simulink model "cascadeHbridge"  (R2024a)
settings: Solver=VariableStepAuto  StartTime=0.0  StopTime=1  RelTol=1e-3
libraries: spsIGBTDiodeLib x24, spsTriangleGeneratorLib x12, spsDCVoltageSourceLib x6, spsSeriesRLCBranchLib x3, spsGroundLib x2, spsThreePhaseVIMeasurementLib x1, sps_lib x1
settings Model: Creator=SAI DEEPAK  LastModifiedBy=SAI DEEPAK
settings DataIOCC: ReturnWorkspaceOutputs=off

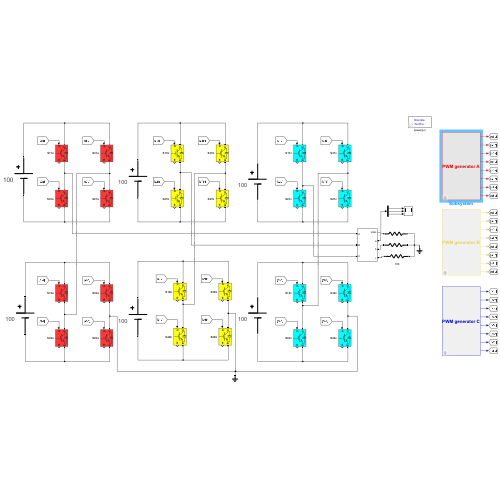
[thumbnail: Simulink's stored preview of the top-level diagram]
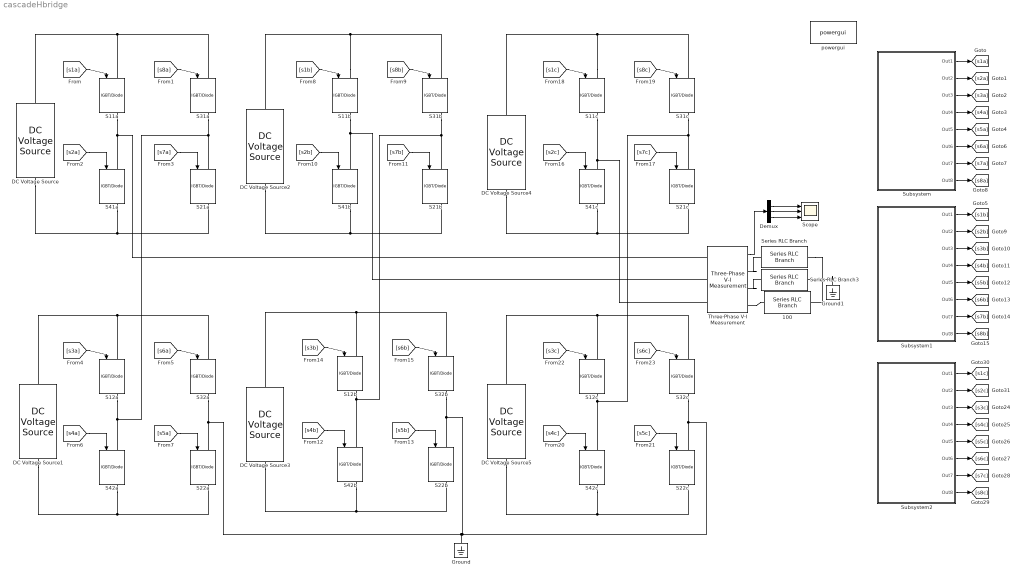
== system cascadeHbridge ==
  100 : spsSeriesRLCBranchLib/Series RLC Branch  LConnTagsString=__new0  RConnTagsString=__new0  BranchType=R  Resistance=100  Inductance=1e-3  SetiL0=off  InitialCurrent=0  Capacitance=1e-6  Setx0=off  InitialVoltage=0  Measurements=None
  DC Voltage Source{,1..5} (6 alike) : spsDCVoltageSourceLib/DC Voltage Source  Amplitude=100  Measurements=None
      settings: AttributesFormatString=%<Amplitude>
  Demux : Demux  Outputs=3
  Ground : spsGroundLib/Ground  LConnTagsString=a
  Ground1 : spsGroundLib/Ground  LConnTagsString=a
  S11a : spsIGBTDiodeLib/IGBT//Diode  Ron=1e-3  Rs=1e5  Cs=inf  Measurements=on
  S11b : spsIGBTDiodeLib/IGBT//Diode  Ron=1e-3  Rs=1e5  Cs=inf  Measurements=on
  S11c : spsIGBTDiodeLib/IGBT//Diode  Ron=1e-3  Rs=1e5  Cs=inf  Measurements=on
  S12a : spsIGBTDiodeLib/IGBT//Diode  Ron=1e-3  Rs=1e5  Cs=inf  Measurements=on
  S12b : spsIGBTDiodeLib/IGBT//Diode  Ron=1e-3  Rs=1e5  Cs=inf  Measurements=on
  S12c : spsIGBTDiodeLib/IGBT//Diode  Ron=1e-3  Rs=1e5  Cs=inf  Measurements=on
  S21a : spsIGBTDiodeLib/IGBT//Diode  Ron=1e-3  Rs=1e5  Cs=inf  Measurements=on
  S21b : spsIGBTDiodeLib/IGBT//Diode  Ron=1e-3  Rs=1e5  Cs=inf  Measurements=on
  S21c : spsIGBTDiodeLib/IGBT//Diode  Ron=1e-3  Rs=1e5  Cs=inf  Measurements=on
  S22a : spsIGBTDiodeLib/IGBT//Diode  Ron=1e-3  Rs=1e5  Cs=inf  Measurements=on
  S22b : spsIGBTDiodeLib/IGBT//Diode  Ron=1e-3  Rs=1e5  Cs=inf  Measurements=on
  S22c : spsIGBTDiodeLib/IGBT//Diode  Ron=1e-3  Rs=1e5  Cs=inf  Measurements=on
  S31a : spsIGBTDiodeLib/IGBT//Diode  Ron=1e-3  Rs=1e5  Cs=inf  Measurements=on
  S31b : spsIGBTDiodeLib/IGBT//Diode  Ron=1e-3  Rs=1e5  Cs=inf  Measurements=on
  S31c : spsIGBTDiodeLib/IGBT//Diode  Ron=1e-3  Rs=1e5  Cs=inf  Measurements=on
  S32a : spsIGBTDiodeLib/IGBT//Diode  Ron=1e-3  Rs=1e5  Cs=inf  Measurements=on
  S32b : spsIGBTDiodeLib/IGBT//Diode  Ron=1e-3  Rs=1e5  Cs=inf  Measurements=on
  S32c : spsIGBTDiodeLib/IGBT//Diode  Ron=1e-3  Rs=1e5  Cs=inf  Measurements=on
  S41a : spsIGBTDiodeLib/IGBT//Diode  Ron=1e-3  Rs=1e5  Cs=inf  Measurements=on
  S41b : spsIGBTDiodeLib/IGBT//Diode  Ron=1e-3  Rs=1e5  Cs=inf  Measurements=on
  S41c : spsIGBTDiodeLib/IGBT//Diode  Ron=1e-3  Rs=1e5  Cs=inf  Measurements=on
  S42a : spsIGBTDiodeLib/IGBT//Diode  Ron=1e-3  Rs=1e5  Cs=inf  Measurements=on
  S42b : spsIGBTDiodeLib/IGBT//Diode  Ron=1e-3  Rs=1e5  Cs=inf  Measurements=on
  S42c : spsIGBTDiodeLib/IGBT//Diode  Ron=1e-3  Rs=1e5  Cs=inf  Measurements=on
  Scope : Scope  NumInputPorts=3
  Series RLC Branch : spsSeriesRLCBranchLib/Series RLC Branch  LConnTagsString=__new0  RConnTagsString=__new0  BranchType=R  Resistance=100  Inductance=1e-3  SetiL0=off  InitialCurrent=0  Capacitance=1e-6  Setx0=off  InitialVoltage=0  Measurements=None
  Series RLC Branch3 : spsSeriesRLCBranchLib/Series RLC Branch  LConnTagsString=__new0  RConnTagsString=__new0  BranchType=R  Resistance=100  Inductance=1e-3  SetiL0=off  InitialCurrent=0  Capacitance=1e-6  Setx0=off  InitialVoltage=0  Measurements=None
  Subsystem : Subsystem  mask{Amplitude=0.8, Frequency=2*pi*50, Phaseangle=0, Freq1=2e3, Phase1=0, Freq2=2e3, Phase2=270, Freq3=2e3, Phase3=180, Freq4=2e3, Phase4=90}
      mask prompts: Amplitude "Simulink:blkprm_prompts:SinWaveAmplitude"; Frequency "Simulink:blkprm_prompts:SinWaveFrequency"; Phaseangle "Simulink:blkprm_prompts:SinWavePhase"; Freq1 "Frequency (Hz):"; Phase1 "Phase (degrees):"; Freq2 "Frequency (Hz):"; Phase2 "Phase (degrees):"; Freq3 "Frequency (Hz):"; Phase3 "Phase (degrees):"; Freq4 "Frequency (Hz):"; Phase4 "Phase (degrees):"
      mask TypeOptions Amplitude: Sine Wave/Amplitude
      mask TypeOptions Frequency: Sine Wave/Frequency
      mask TypeOptions Phaseangle: Sine Wave/Phase
      mask TypeOptions Freq1:
      | Triangle
      | Generator1/Freq
      mask TypeOptions Phase1:
      | Triangle
      | Generator1/Phase
      mask TypeOptions Freq2:
      | Triangle
      | Generator2/Freq
      mask TypeOptions Phase2:
      | Triangle
      | Generator2/Phase
      mask TypeOptions Freq3:
      | Triangle
      | Generator3/Freq
      mask TypeOptions Phase3:
      | Triangle
      | Generator3/Phase
      mask TypeOptions Freq4:
      | Triangle
      | Generator4/Freq
      mask TypeOptions Phase4:
      | Triangle
      | Generator4/Phase
      mask DialogControl Sinewave Prompt: (Add text here)
      mask DialogControl Amplitude Prompt: Amplitude:
      mask DialogControl Frequency Prompt: Frequency (rad/sec):
      mask DialogControl Phaseangle Prompt: Phase (rad):
      mask DialogControl carriersignal1 Prompt: (Add text here)
      mask DialogControl carriersignal2 Prompt: (Add text here)
      mask DialogControl carriersignal3 Prompt: (Add text here)
      mask DialogControl carriersignal4 Prompt: (Add text here)
      mask Display:
      | color('red');
      | disp('PWM generator A');
  Subsystem1 : Subsystem  mask{Amplitude=0.8, Frequency=2*pi*50, Phase=-2*pi/3, Freq1=2e3, Phase1=0, Freq2=2e3, Phase2=270, Freq3=2e3, Phase3=180, Freq4=2e3, Phase4=90}
      mask prompts: Amplitude "Simulink:blkprm_prompts:SinWaveAmplitude"; Frequency "Simulink:blkprm_prompts:SinWaveFrequency"; Phase "Simulink:blkprm_prompts:SinWavePhase"; Freq1 "Frequency (Hz):"; Phase1 "Phase (degrees):"; Freq2 "Frequency (Hz):"; Phase2 "Phase (degrees):"; Freq3 "Frequency (Hz):"; Phase3 "Phase (degrees):"; Freq4 "Frequency (Hz):"; Phase4 "Phase (degrees):"
      mask TypeOptions Amplitude: Sine Wave1/Amplitude
      mask TypeOptions Frequency: Sine Wave1/Frequency
      mask TypeOptions Phase: Sine Wave1/Phase
      mask TypeOptions Freq1:
      | Triangle
      | Generator4/Freq
      mask TypeOptions Phase1:
      | Triangle
      | Generator4/Phase
      mask TypeOptions Freq2:
      | Triangle
      | Generator5/Freq
      mask TypeOptions Phase2:
      | Triangle
      | Generator5/Phase
      mask TypeOptions Freq3:
      | Triangle
      | Generator6/Freq
      mask TypeOptions Phase3:
      | Triangle
      | Generator6/Phase
      mask TypeOptions Freq4:
      | Triangle
      | Generator7/Freq
      mask TypeOptions Phase4:
      | Triangle
      | Generator7/Phase
      mask DialogControl Control6 Prompt: modulating signal
      mask DialogControl Amplitude Prompt: Amplitude:
      mask DialogControl Frequency Prompt: Frequency (rad/sec):
      mask DialogControl Phase Prompt: Phase (rad):
      mask DialogControl Control1 Prompt: carrier signal 1
      mask DialogControl Control4 Prompt: carrier signal 2
      mask DialogControl Control3 Prompt: carrier signal 3
      mask DialogControl Control2 Prompt: carrier signal 4
      mask Display:
      | color('yellow');
      | disp('PWM generator B');
  Subsystem2 : Subsystem  mask{Amplitude=0.8, Frequency=2*pi*50, Phase=2*pi/3, Freq1=2e3, Phase1=0, Phase2=90, Freq2=2e3, Freq3=2e3, Phase3=180, Phase4=270, Freq4=2e3}
      mask prompts: Amplitude "Simulink:blkprm_prompts:SinWaveAmplitude"; Frequency "Simulink:blkprm_prompts:SinWaveFrequency"; Phase "Simulink:blkprm_prompts:SinWavePhase"; Freq1 "Frequency (Hz):"; Phase1 "Phase (degrees):"; Phase2 "Phase (degrees):"; Freq2 "Frequency (Hz):"; Freq3 "Frequency (Hz):"; Phase3 "Phase (degrees):"; Phase4 "Phase (degrees):"; Freq4 "Frequency (Hz):"
      mask TypeOptions Amplitude: Sine Wave3/Amplitude
      mask TypeOptions Frequency: Sine Wave3/Frequency
      mask TypeOptions Phase: Sine Wave3/Phase
      mask TypeOptions Freq1:
      | Triangle
      | Generator14/Freq
      mask TypeOptions Phase1:
      | Triangle
      | Generator14/Phase
      mask TypeOptions Phase2:
      | Triangle
      | Generator13/Phase
      mask TypeOptions Freq2:
      | Triangle
      | Generator13/Freq
      mask TypeOptions Freq3:
      | Triangle
      | Generator12/Freq
      mask TypeOptions Phase3:
      | Triangle
      | Generator12/Phase
      mask TypeOptions Phase4:
      | Triangle
      | Generator15/Phase
      mask TypeOptions Freq4:
      | Triangle
      | Generator15/Freq
      mask DialogControl Control2 Prompt: modulating signal
      mask DialogControl Amplitude Prompt: Amplitude:
      mask DialogControl Frequency Prompt: Frequency (rad/sec):
      mask DialogControl Phase Prompt: Phase (rad):
      mask DialogControl Control4 Prompt: carrier signal 1
      mask DialogControl Control5 Prompt: carrier signal 2
      mask DialogControl Control3 Prompt: carrier signal3
      mask DialogControl Control6 Prompt: carrier signal4
      mask Display:
      | color('blue');
      | disp('PWM generator C');
  Three-Phase V-I Measurement : spsThreePhaseVIMeasurementLib/Three-Phase V-I Measurement  VoltageMeasurement=phase-to-ground  SetLabelV=off  LabelV=Vabc  Vpu=off  VpuLL=off  CurrentMeasurement=no  SetLabelI=off  LabelI=Iabc  Ipu=off  Pbase=100e6  Vbase=500e3  OutputType=Complex  PhasorSimulation=off  PSBequivalent=0
  powergui : sps_lib/powergui  Priority=1  SimulationMode=Discrete  SampleTime=5e-6  frequency=60  Iterations=50  frequencyindice=0  Pbase=100e6  ErrMax=1e-4  UnitsV=kV  UnitsW=MW  buscounter=0  FunctionMessages=off  echomessages=off  EnableUseOfTLC=off  CurrentSourceSwitches=off  DisableSnubberDevices=off  DisableRonSwitches=off  DisableVfSwitches=off  DisplayEquations=off  AutomaticDiscreteSolvers=off  SolverType=Tustin/Backward Euler (TBE)  Interpol=off  ExternalGateDelay=off  methode=off  Ts=100  x0status=blocks  SPID=on  SwTol=0  HookPort=off  NonlinearTolerance=1e-4  nMaxIteration=100  ContinueOnMaxIteration=off  RestoreLinks=warning  ResistiveCurrentMeasurement=off  Frange=[0:2:500]  Ylog=off  Xlog=on  ShowGrid=off  save=off  variable=ZData  structure=0  ZoomFFT=off  StartTime=0.0  cycles=1  DisplayStyle=1  fundamental=60  FreqAxis=off  MaxFrequency=1000  frequencyindicesteady=1  RmsSteady=1  display=off
  wires:
  [s1a] -> S11a/1
  [s2a] -> S41a/1
  [s8a] -> S31a/1
  [s7a] -> S21a/1
  [s3a] -> S12a/1
  [s4a] -> S42a/1
  [s6a] -> S32a/1
  [s5a] -> S22a/1
  [s1b] -> S11b/1
  [s2b] -> S41b/1
  [s8b] -> S31b/1
  [s7b] -> S21b/1
  [s6b] -> S32b/1
  [s3b] -> S12b/1
  [s4b] -> S42b/1
  [s5b] -> S22b/1
  [s1c] -> S11c/1
  [s2c] -> S41c/1
  [s8c] -> S31c/1
  [s7c] -> S21c/1
  [s3c] -> S12c/1
  [s4c] -> S42c/1
  [s6c] -> S32c/1
  [s5c] -> S22c/1
  Subsystem/1(Out1) -> [s1a]
  Subsystem/2(Out2) -> [s2a]
  Subsystem/3(Out3) -> [s3a]
  Subsystem/4(Out4) -> [s4a]
  Subsystem/5(Out5) -> [s5a]
  Subsystem/6(Out6) -> [s6a]
  Subsystem/7(Out7) -> [s7a]
  Subsystem/8(Out8) -> [s8a]
  Subsystem1/1(Out1) -> [s1b]
  Subsystem1/2(Out2) -> [s2b]
  Subsystem1/3(Out3) -> [s3b]
  Subsystem1/4(Out4) -> [s4b]
  Subsystem1/5(Out5) -> [s5b]
  Subsystem1/6(Out6) -> [s6b]
  Subsystem1/7(Out7) -> [s7b]
  Subsystem1/8(Out8) -> [s8b]
  Subsystem2/1(Out1) -> [s1c]
  Subsystem2/2(Out2) -> [s2c]
  Subsystem2/3(Out3) -> [s3c]
  Subsystem2/4(Out4) -> [s4c]
  Subsystem2/5(Out5) -> [s5c]
  Subsystem2/6(Out6) -> [s6c]
  Subsystem2/7(Out7) -> [s7c]
  Subsystem2/8(Out8) -> [s8c]
  Three-Phase V-I Measurement/1 -> Demux/1
  Demux/1 -> Scope/1
  Demux/2 -> Scope/2
  Demux/3 -> Scope/3
  connections:
  S41a/RConn1 -- DC Voltage Source/LConn1 -- S21a/RConn1
  S31a/LConn1 -- DC Voltage Source/RConn1 -- S11a/LConn1
  S11a/RConn1 -- Three-Phase V-I Measurement/LConn1 -- S41a/LConn1
  S42a/RConn1 -- DC Voltage Source1/LConn1 -- S22a/RConn1
  S32a/LConn1 -- DC Voltage Source1/RConn1 -- S12a/LConn1
  S12a/RConn1 -- S31a/RConn1 -- S21a/LConn1 -- S42a/LConn1
  S41b/RConn1 -- DC Voltage Source2/LConn1 -- S21b/RConn1
  S11b/LConn1 -- DC Voltage Source2/RConn1 -- S31b/LConn1
  S11b/RConn1 -- S41b/LConn1 -- Three-Phase V-I Measurement/LConn2
  S42b/RConn1 -- DC Voltage Source3/LConn1 -- S22b/RConn1
  S32b/LConn1 -- DC Voltage Source3/RConn1 -- S12b/LConn1
  S12b/RConn1 -- S42b/LConn1 -- S31b/RConn1 -- S21b/LConn1
  S41c/RConn1 -- DC Voltage Source4/LConn1 -- S21c/RConn1
  S11c/LConn1 -- DC Voltage Source4/RConn1 -- S31c/LConn1
  S11c/RConn1 -- Three-Phase V-I Measurement/LConn3 -- S41c/LConn1
  S42c/RConn1 -- DC Voltage Source5/LConn1 -- S22c/RConn1
  S32c/LConn1 -- DC Voltage Source5/RConn1 -- S12c/LConn1
  S32c/RConn1 -- Ground/LConn1 -- S32a/RConn1 -- S22a/LConn1 -- S32b/RConn1 -- S22b/LConn1 -- S22c/LConn1
  S12c/RConn1 -- S42c/LConn1 -- S31c/RConn1 -- S21c/LConn1
  Three-Phase V-I Measurement/RConn1 -- Series RLC Branch/LConn1
  Three-Phase V-I Measurement/RConn2 -- Series RLC Branch3/LConn1
  Three-Phase V-I Measurement/RConn3 -- 100/LConn1
  Series RLC Branch/RConn1 -- 100/RConn1 -- Ground1/LConn1 -- Series RLC Branch3/RConn1

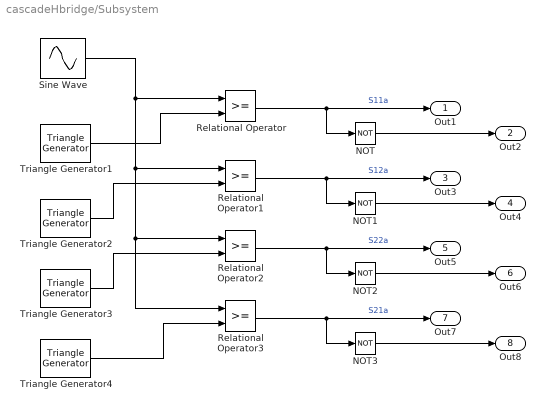
== system cascadeHbridge/Subsystem ==
  NOT{,1..3} (4 alike) : Logic  Operator=NOT  IconShape=distinctive  AllPortsSameDT=off  OutDataTypeStr=boolean
  Relational Operator{,1..3} (4 alike) : RelationalOperator  OutDataTypeStr=boolean  RndMeth=Simplest  InputSameDT=off
  Sine Wave : Sin  Amplitude=Amplitude  Frequency=Frequency  Phase=Phaseangle  SampleTime=0
  Triangle Generator1 : spsTriangleGeneratorLib/Triangle Generator  Freq=Freq1  Phase=Phase1  Ts=0
  Triangle Generator2 : spsTriangleGeneratorLib/Triangle Generator  Freq=Freq2  Phase=Phase2  Ts=0
  Triangle Generator3 : spsTriangleGeneratorLib/Triangle Generator  Freq=Freq3  Phase=Phase3  Ts=0
  Triangle Generator4 : spsTriangleGeneratorLib/Triangle Generator  Freq=Freq4  Phase=Phase4  Ts=0
  Out1 : Outport
  Out2 : Outport  Port=2
  Out3 : Outport  Port=3
  Out4 : Outport  Port=4
  Out5 : Outport  Port=5
  Out6 : Outport  Port=6
  Out7 : Outport  Port=7
  Out8 : Outport  Port=8
  wires:
  Relational Operator/1 -> Out1/1, NOT/1  "S11a"
  Triangle Generator1/1 -> Relational Operator/2
  Triangle Generator3/1 -> Relational Operator2/2
  Relational Operator1/1 -> Out3/1, NOT1/1  "S12a"
  Relational Operator3/1 -> NOT3/1, Out7/1  "S21a"
  Relational Operator2/1 -> Out5/1, NOT2/1  "S22a"
  Triangle Generator4/1 -> Relational Operator3/2
  Sine Wave/1 -> Relational Operator/1, Relational Operator1/1, Relational Operator3/1, Relational Operator2/1
  Triangle Generator2/1 -> Relational Operator1/2
  NOT2/1 -> Out6/1
  NOT1/1 -> Out4/1
  NOT3/1 -> Out8/1
  NOT/1 -> Out2/1

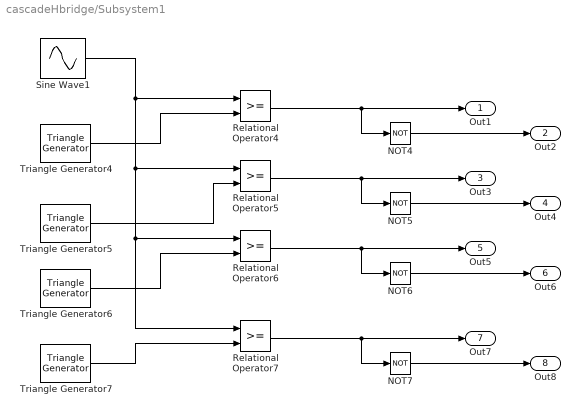
== system cascadeHbridge/Subsystem1 ==
  NOT{4..7} (4 alike) : Logic  Operator=NOT  IconShape=distinctive  AllPortsSameDT=off  OutDataTypeStr=boolean
  Relational Operator{4..7} (4 alike) : RelationalOperator  OutDataTypeStr=boolean  RndMeth=Simplest  InputSameDT=off
  Sine Wave1 : Sin  Amplitude=Amplitude  Frequency=Frequency  Phase=Phase  SampleTime=0
  Triangle Generator4 : spsTriangleGeneratorLib/Triangle Generator  Freq=Freq1  Phase=Phase1  Ts=0
  Triangle Generator5 : spsTriangleGeneratorLib/Triangle Generator  Freq=Freq2  Phase=Phase2  Ts=0
  Triangle Generator6 : spsTriangleGeneratorLib/Triangle Generator  Freq=Freq3  Phase=Phase3  Ts=0
  Triangle Generator7 : spsTriangleGeneratorLib/Triangle Generator  Freq=Freq4  Phase=Phase4  Ts=0
  Out1 : Outport
  Out2 : Outport  Port=2
  Out3 : Outport  Port=3
  Out4 : Outport  Port=4
  Out5 : Outport  Port=5
  Out6 : Outport  Port=6
  Out7 : Outport  Port=7
  Out8 : Outport  Port=8
  wires:
  NOT5/1 -> Out4/1
  Relational Operator6/1 -> Out5/1, NOT6/1
  Triangle Generator6/1 -> Relational Operator6/2
  Triangle Generator5/1 -> Relational Operator5/2
  Sine Wave1/1 -> Relational Operator5/1, Relational Operator7/1, Relational Operator6/1, Relational Operator4/1
  Relational Operator7/1 -> Out7/1, NOT7/1
  Triangle Generator7/1 -> Relational Operator7/2
  Relational Operator5/1 -> Out3/1, NOT5/1
  Relational Operator4/1 -> Out1/1, NOT4/1
  NOT6/1 -> Out6/1
  Triangle Generator4/1 -> Relational Operator4/2
  NOT7/1 -> Out8/1
  NOT4/1 -> Out2/1

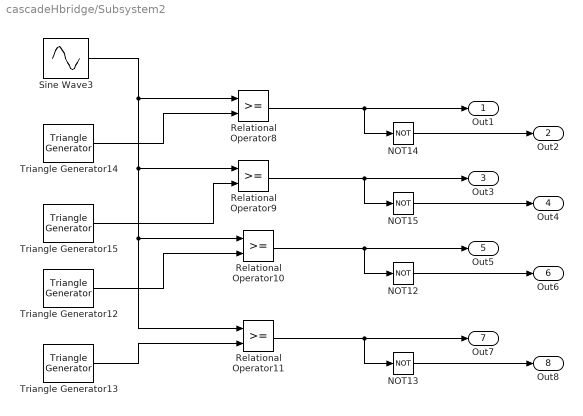
== system cascadeHbridge/Subsystem2 ==
  NOT{12..15} (4 alike) : Logic  Operator=NOT  IconShape=distinctive  AllPortsSameDT=off  OutDataTypeStr=boolean
  Relational Operator{8..11} (4 alike) : RelationalOperator  OutDataTypeStr=boolean  RndMeth=Simplest  InputSameDT=off
  Sine Wave3 : Sin  Amplitude=Amplitude  Frequency=Frequency  Phase=Phase  SampleTime=0
  Triangle Generator12 : spsTriangleGeneratorLib/Triangle Generator  Freq=Freq3  Phase=Phase3  Ts=0
  Triangle Generator13 : spsTriangleGeneratorLib/Triangle Generator  Freq=Freq2  Phase=Phase2  Ts=0
  Triangle Generator14 : spsTriangleGeneratorLib/Triangle Generator  Freq=Freq1  Phase=Phase1  Ts=0
  Triangle Generator15 : spsTriangleGeneratorLib/Triangle Generator  Freq=Freq4  Phase=Phase4  Ts=0
  Out1 : Outport
  Out2 : Outport  Port=2
  Out3 : Outport  Port=3
  Out4 : Outport  Port=4
  Out5 : Outport  Port=5
  Out6 : Outport  Port=6
  Out7 : Outport  Port=7
  Out8 : Outport  Port=8
  wires:
  Relational Operator8/1 -> Out1/1, NOT14/1
  Triangle Generator15/1 -> Relational Operator9/2
  Relational Operator11/1 -> Out7/1, NOT13/1
  NOT15/1 -> Out4/1
  Sine Wave3/1 -> Relational Operator9/1, Relational Operator11/1, Relational Operator10/1, Relational Operator8/1
  Relational Operator9/1 -> Out3/1, NOT15/1
  Triangle Generator13/1 -> Relational Operator11/2
  Triangle Generator12/1 -> Relational Operator10/2
  Triangle Generator14/1 -> Relational Operator8/2
  Relational Operator10/1 -> Out5/1, NOT12/1
  NOT13/1 -> Out8/1
  NOT12/1 -> Out6/1
  NOT14/1 -> Out2/1
